simulink model "RW_Time_Delay_Analysis_mdl_cont"  (R2025b)
settings: Solver=VariableStepAuto  StartTime=0.0  StopTime=20  RelTol=1e-3
values from neighbouring files (symbols this model uses):
  Kd = 0.95    [RW_Time_Delay_Analysis.m]    (also in RW_Time_Delay_Analysis_Simulink_Params.m; RW_Time_Delay_Analysis_new_implementation.m)
  Ki = 0.1    [RW_Time_Delay_Analysis.m]    (also in RW_Time_Delay_Analysis_Simulink_Params.m; RW_Time_Delay_Analysis_new_implementation.m)
  Kp = 0.8    [RW_Time_Delay_Analysis.m]    (also in RW_Time_Delay_Analysis_Simulink_Params.m; RW_Time_Delay_Analysis_new_implementation.m)
settings Model: Creator=barinmoghimi  LastModifiedBy=barinmoghimi

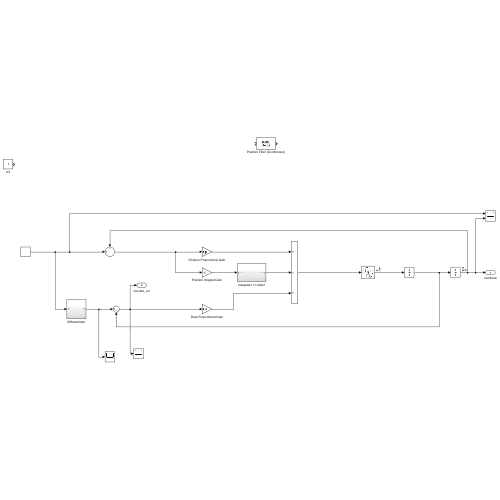
[thumbnail: Simulink's stored preview of the top-level diagram]
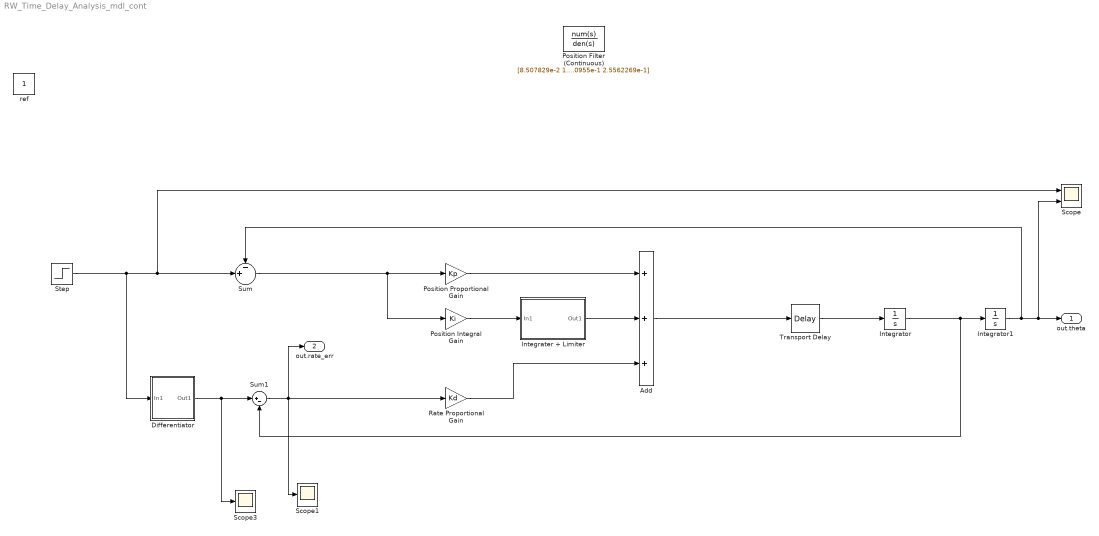
== system RW_Time_Delay_Analysis_mdl_cont ==
  Add : Sum  Inputs=+++
  Differentiator : Subsystem
  Integrater + Limiter : Subsystem
  Integrator : Integrator
  Integrator1 : Integrator
  Position Filter (Continuous) : TransferFcn  Numerator=[8.507829e-2 1.7015657e-1 8.50782e-2]  Denominator=[1.0e+0 -9.1530955e-1 2.5562269e-1]
  Position Integral Gain : Gain  Gain=Ki
  Position Proportional Gain : Gain  Gain=Kp
  Rate Proportional Gain : Gain  Gain=Kd
  Scope : Scope  NumInputPorts=2
      settings: ActiveDisplayYMinimum=-1  ActiveDisplayYMaximum=1
  Scope1 : Scope
      settings: ActiveDisplayYMinimum=-1  ActiveDisplayYMaximum=1
  Scope3 : Scope
      settings: ActiveDisplayYMinimum=-1  ActiveDisplayYMaximum=1  DataLoggingVariableName=ScopeData3
  Step : Step  SampleTime=0
  Sum : Sum  Inputs=-+|
  Sum1 : Sum  Inputs=|+-
  Transport Delay : TransportDelay  DelayTime=50  PadeOrder=5
  ref : Constant
  out.theta : Outport
  out.rate_err : Outport  Port=2
  wires:
  Add/1 -> Transport Delay/1
  Sum/1 -> Position Proportional Gain/1, Position Integral Gain/1
  Position Proportional Gain/1 -> Add/1
  Position Integral Gain/1 -> Integrater + Limiter/1(In1)
  Step/1 -> Differentiator/1(In1), Scope/1, Sum/2
  Differentiator/1(Out1) -> Scope3/1, Sum1/1
  Integrater + Limiter/1(Out1) -> Add/2
  Sum1/1 -> Rate Proportional Gain/1, Scope1/1, out.rate_err/1
  Transport Delay/1 -> Integrator/1
  Rate Proportional Gain/1 -> Add/3
  Integrator/1 -> Integrator1/1, Sum1/2
  Integrator1/1 -> Sum/1, Scope/2, out.theta/1

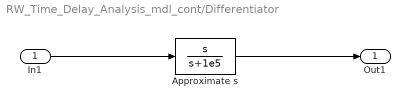
== system RW_Time_Delay_Analysis_mdl_cont/Differentiator ==
  In1 : Inport
  Approximate s : TransferFcn  Numerator=[1 0]  Denominator=[1 1e5]
  Out1 : Outport
  wires:
  Approximate s/1 -> Out1/1
  In1/1 -> Approximate s/1

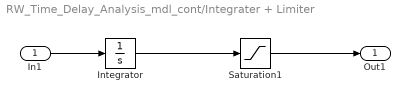
== system RW_Time_Delay_Analysis_mdl_cont/Integrater + Limiter ==
  In1 : Inport
  Integrator : Integrator
  Saturation1 : Saturate  UpperLimit=pi  LowerLimit=-pi
  Out1 : Outport
  wires:
  Integrator/1 -> Saturation1/1
  In1/1 -> Integrator/1
  Saturation1/1 -> Out1/1
